simulink model "Step_1_Observer_Calibration_Experiment"  (R2020a)
settings: Solver=ode4  StartTime=0.0  StopTime=3  FixedStep=1e-6  MaxStep=1e-4  RelTol=1e-3
libraries: fl_lib x5, nesl_utility x5, ee_lib x2, simulink x1, eePwmGenerator x1
settings Model: Creator=nnnmmm  LastModifiedBy=nnnmmm
settings DataIOCC: ExternalInput=sim_input_T

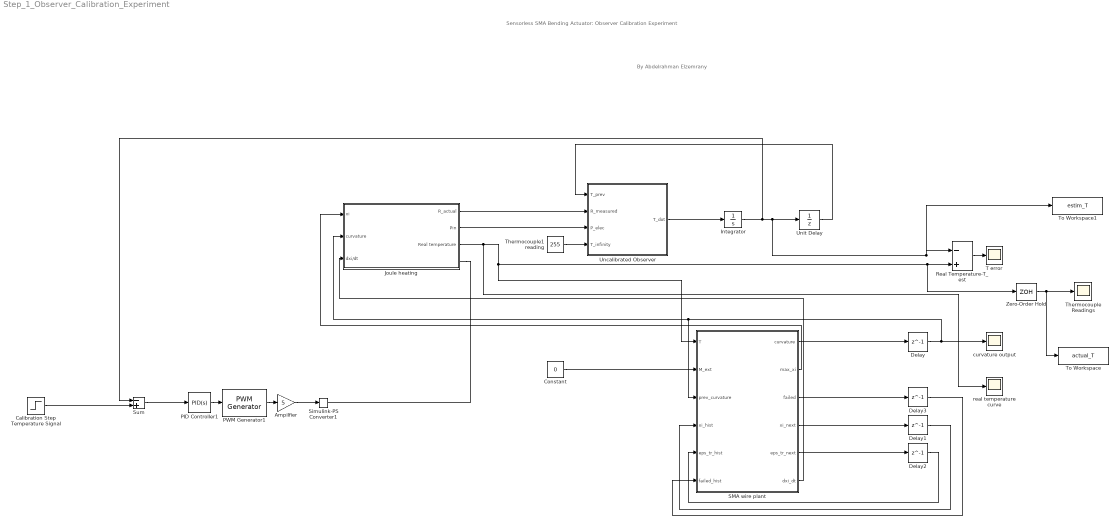
== system Step_1_Observer_Calibration_Experiment ==
  note: By Abdelrahman Elzemrany
  note: Sensorless SMA Bending Actuator: Observer Calibration Experiment
  Ampilfier : Gain  Gain=5
  Calibration Step Temperature Signal : Step  Before=255  After=300  SampleTime=0
  Constant : Constant  Value=0
  Delay : Delay  DelayLength=1
  Delay1 : Delay  DelayLength=1  InitialCondition=ones(1,11)
  Delay2 : Delay  DelayLength=1  InitialCondition=zeros(1,11)
  Delay3 : Delay  DelayLength=1
  Integrator : Integrator  InitialCondition=255
  Joule heating : Subsystem
  PID Controller1 : simulink/Continuous/PID Controller  Controller=PID  Form=Parallel  TimeDomain=Continuous-time  UseExternalTs=off  SampleTime=-1  IntegratorMethod=Forward Euler  FilterMethod=Forward Euler  ControllerParametersSource=internal  P=10  I=5  D=0  UseFilter=on  N=100  TunerSelectOption=Transfer Function Based (PID Tuner App)  InitialConditionSource=internal  InitialConditionForIntegrator=0  InitialConditionForFilter=0  DifferentiatorICPrevScaledInput=0  ExternalReset=none  TrackingMode=off  Kt=1  LimitOutput=on  UpperSaturationLimit=1  LowerSaturationLimit=0  LinearizeAsGain=on  AntiWindupMode=clamping  Kb=1  POutMin=[]  POutMax=[]  IOutMin=[]  IOutMax=[]  DOutMin=[]  DOutMax=[]  NOutMin=[]  NOutMax=[]  SumOutMin=[]  SumOutMax=[]  SaturationOutMin=[]  SaturationOutMax=[]  PParamMin=[]  PParamMax=[]  IParamMin=[]  IParamMax=[]  DParamMin=[]  DParamMax=[]  NParamMin=[]  NParamMax=[]  KbParamMin=[]  KbParamMax=[]  KtParamMin=[]  KtParamMax=[]  KbOutMin=[]  KbOutMax=[]  KtOutMin=[]  KtOutMax=[]  IntegratorOutMin=[]  IntegratorOutMax=[]  FilterOutMin=[]  FilterOutMax=[]  SumI1OutMin=[]  SumI1OutMax=[]  SumI2OutMin=[]  SumI2OutMax=[]  SumI3OutMin=[]  SumI3OutMax=[]  SumI4OutMin=[]  SumI4OutMax=[]  SumDOutMin=[]  SumDOutMax=[]  DifferentiatorOutMin=[]  DifferentiatorOutMax=[]  FilterDiffOutCoefMin=[]  FilterDiffOutCoefMax=[]  ReciprocalOutMin=[]  ReciprocalOutMax=[]  SumDenOutMin=[]  SumDenOutMax=[]  SumNumOutMin=[]  SumNumOutMax=[]  DivideOutMin=[]  DivideOutMax=[]  UdiffTsProdOutMin=[]  UdiffTsProdOutMax=[]  NTsProdOutMin=[]  NTsProdOutMax=[]  UintegralTsProdOutMin=[]  UintegralTsProdOutMax=[]  UngainTsProdOutMin=[]  UngainTsProdOutMax=[]  IntegratorContinuousStateAttributes=''  IntegratorStateMustResolveToSignalObject=off  IntegratorRTWStateStorageClass=Auto  FilterContinuousStateAttributes=''  FilterStateMustResolveToSignalObject=off  FilterRTWStateStorageClass=Auto  ParallelPVariant=InternalParameters  IdealPVariant=Disabled  IVariant=InternalParameters  DVariant=InternalParameters  IntegratorVariant=Continuous  SatVariant=Enabled  AWVariant=ContClampingParallel  PCopyVariant=Disabled  TRVariant=Disabled  FdbkBlocksVariant=Forward  IdealPFdbkVariant=Disabled  SatFdbkVariant=Disabled  DerivativeFilterVariant=ContFilter  NVariant=InternalParameters  NCopyVariant=Disabled  FilterICVariant=InternalICsFilter  IntegratorICVariant=InternalICs  ExternalResetVariant=Disabled  TRSumVariant=Passthrough  SumFdbkVariant=Disabled  SumVariant=Sum_PID  TsampFilterVariant=InternalTs  TsampNgainVariant=Passthrough  TsampIntegralVariant=Passthrough
  PWM Generator1 : eePwmGenerator/PWM Generator  CarrCount=Up  Tper=.00001  Ts=1e-6
  Real Temperature-T_est : Sum  Inputs=|-+
  SMA wire plant : MATLAB Function  TreatAsAtomicUnit=on
  Simulink-PS Converter1 : nesl_utility/Simulink-PS Converter  PhysicalDomain=network_engine_domain  SubClassName=ps_input  LeftPortType=input  RightPortType=output  PseudoPeriodic=off  Frequencies=[]  NoiseDistribution=none  NoiseParameters=[]  Unit=1  AffineConversion=off  FilteringAndDerivatives=filter  SimscapeFilterOrder=1  InputFilterTimeConstant=1e-6  UdotUserProvided=0
  Sum : Sum  Inputs=-+
  T error : Scope
  Thermocouple Readings : Scope
  Thermocouple1 reading : Constant  Value=255
  To Workspace : ToWorkspace  VariableName=actual_T  SaveFormat=Timeseries  SampleTime=.230
  To Workspace1 : ToWorkspace  VariableName=estim_T  SaveFormat=Timeseries  SampleTime=.001
  Uncalibrated Observer : MATLAB Function  TreatAsAtomicUnit=on
  Unit Delay : UnitDelay  SampleTime=-1  HasFrameUpgradeWarning=on
  Zero-Order Hold : ZeroOrderHold  SampleTime=.230
  curvature output : Scope
  real temperature curve : Scope
  wires:
  Delay2/1 -> SMA wire plant/5(eps_tr_hist)
  SMA wire plant/5(eps_tr_next) -> Delay2/1
  SMA wire plant/1(curvature) -> Delay/1
  SMA wire plant/3(failed) -> Delay3/1
  SMA wire plant/4(xi_next) -> Delay1/1
  Delay/1 -> curvature output/1, Joule heating/2(curvature), SMA wire plant/3(prev_curvature)
  Delay3/1 -> SMA wire plant/6(failed_hist)
  Delay1/1 -> SMA wire plant/4(xi_hist)
  Constant/1 -> SMA wire plant/2(M_ext)
  SMA wire plant/2(max_xi) -> Joule heating/1(xi)
  SMA wire plant/6(dxi_dt) -> Joule heating/3(dxi/dt)
  PWM Generator1/1 -> Ampilfier/1
  PID Controller1/1 -> PWM Generator1/1
  Ampilfier/1 -> Simulink-PS Converter1/1
  Joule heating/2(Pin) -> Uncalibrated Observer/3(P_elec)
  Joule heating/1(R_actual) -> Uncalibrated Observer/2(R_measured)
  Uncalibrated Observer/1(T_dot) -> Integrator/1
  Integrator/1 -> Sum/1, Unit Delay/1, To Workspace1/1, Real Temperature-T_est/1
  Thermocouple1 reading/1 -> Uncalibrated Observer/4(T_infinity)
  Joule heating/3(Real temperature) -> real temperature curve/1, SMA wire plant/1(T), Zero-Order Hold/1, Real Temperature-T_est/2
  Real Temperature-T_est/1 -> T error/1
  Unit Delay/1 -> Uncalibrated Observer/1(T_prev)
  Sum/1 -> PID Controller1/1
  Calibration Step Temperature Signal/1 -> Sum/2
  Zero-Order Hold/1 -> To Workspace/1, Thermocouple Readings/1
  connections:
  Joule heating/RConn1 -- Simulink-PS Converter1/RConn1

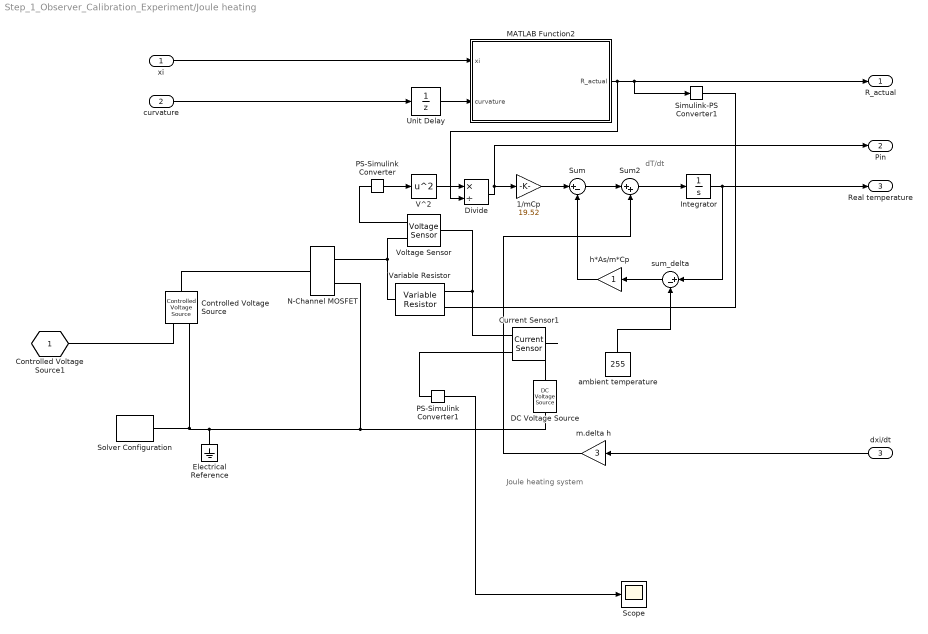
== system Step_1_Observer_Calibration_Experiment/Joule heating ==
  note: Joule heating system
  note: dT/dt
  xi : Inport
  curvature : Inport  Port=2
  dxi/dt : Inport  Port=3
  1/mCp : Gain  Gain=19.52
  Controlled Voltage Source : fl_lib/Electrical/Electrical Sources/Controlled Voltage Source
  Current Sensor1 : fl_lib/Electrical/Electrical Sensors/Current Sensor
  DC Voltage Source : ee_lib/Additional Components/SPICE Sources/DC Voltage Source  DC=2 V
  Divide : Product  Inputs=*/
  Electrical Reference : fl_lib/Electrical/Electrical Elements/Electrical Reference
      settings: SourceProductBaseCode=MT,SS
  Integrator : Integrator  InitialCondition=255
  MATLAB Function2 : MATLAB Function  TreatAsAtomicUnit=on
  N-Channel MOSFET : ee_lib/Semiconductors & Converters/N-Channel MOSFET  paramTerminal=ee.enum.mosfet.numberOfTerminals.three  parameterization=ee.enum.parameterization.datasheet  prmDatasheet=ee.enum.temperatureParameterization.none  prmEquCoeff=ee.enum.temperatureParameterization.none  Beta=5.0 A/V^2  Rds=0.010 Ohm  Id=6.0 A  Vgs=10 V  Vth=1.7 V  Vth0=1.7 V  lam=0 1/V  gamma_vth=0.5 V^0.50000  phib=0.5 V  Vth1=1.9071 V  Vbs1=-1 V  Vth2=2.066 V  Vbs2=-2 V  Tmeas=25 degC  RS=0.0001 Ohm  RD=1e-4 Ohm  RB=0.001 Ohm  C_param=ee.enum.mosfet.capacitanceParam.fixedciss  C_GS=270 pF  C_GD=80 pF  C_DS=0 pF  C_iss=350 pF  C_rss=80 pF  C_oss=0 pF  charge_linearity_param=ee.enum.mosfet.cgdLinearity.constant  C_OX=200 pF  V_C_OX=-0.5 V  C_iss_vec=[720, 700, 590, 470, 390, 310] pF  C_rss_vec=[450, 400, 300, 190, 95, 55] pF  C_oss_vec=[900, 810, 690, 420, 270, 170] pF  C_GS_vec=[270, 300, 290, 280, 295, 255] pF  C_GD_vec=[450, 400, 300, 190, 95, 55] pF  C_DS_vec=[450, 410, 390, 230, 175, 115] pF  C_Vds_vec=[.1, .3, 1, 3, 10, 30] V  V_GS_for_cap_data=0 V  charge_linearity_param_vgb=ee.enum.mosfet.cgbLinearity.instantly  IsDiode=0 A  Vbi=0.6 V  n=1  Cj0Diode=0 pF  TT=50e-9 s  dVth_dT=-6 mV/K  dVth0_dT=-6 mV/K  Rds_T2=0.037 Ohm  Tmeas2=125 degC  BEXDatasheet=-1.5  BEXEquCoeff=-1.5  etaisDatasheet=3  etaisEquCoeff=3  TdeviceDatasheet=25 degC  TdeviceEquCoeff=25 degC  thermal_network_parameterization=ee.enum.thermalNetworkTopology.cauer  Rth=[0, 10] K/W  Rth_Foster=[4, 6] K/W  thermal_mass_parameterization=ee.enum.thermalNetwork.timeconstant  thermal_mass=[0, 1] J/K  thermal_mass_Foster=[1.5, 3] J/K  thermal_time_constant=[0, 10] s  thermal_time_constant_Foster=[6, 18] s  thermal_mass_initial_temperatures=[25, 25] degC  betaref=18 A/V^2  Vfbref=-1.1 V  gamma=3.5 V^0.50000  phib2ref=1 V  thesatref=0.4 1/V  alpha=0  Vp=5e-2 V  thesrref=0 1/V  m=8  Tref=25 degC  Cox=1500 pF  Cgso=100 pF  Cgdo=14 pF  Rsref=2e-3 Ohm  Rdref=0.17 Ohm  Rgref=8.4 Ohm  Rbref=2e-3 Ohm  Isref=5.2e-13 A  Cj0=480 pF  Tprm=1  etabet=1.3  Stvfb=5e-4 V/K  Stphib=-8.5e-4 V/K  etasat=1.04  etasr=0.65  etar=0.95  etais=3  Tsim=25 degC  T0=[25, 25] degC
  PS-Simulink Converter : nesl_utility/PS-Simulink Converter  PhysicalDomain=network_engine_domain  SubClassName=ps_output  LeftPortType=input  RightPortType=output  PseudoPeriodic=off  Frequencies=[]  Unit=inherit  AffineConversion=off
  PS-Simulink Converter1 : nesl_utility/PS-Simulink Converter  PhysicalDomain=network_engine_domain  SubClassName=ps_output  LeftPortType=input  RightPortType=output  PseudoPeriodic=off  Frequencies=[]  Unit=inherit  AffineConversion=off
  Scope : Scope
  Simulink-PS Converter1 : nesl_utility/Simulink-PS Converter  PhysicalDomain=network_engine_domain  SubClassName=ps_input  LeftPortType=input  RightPortType=output  PseudoPeriodic=off  Frequencies=[]  NoiseDistribution=none  NoiseParameters=[]  Unit=1  AffineConversion=off  FilteringAndDerivatives=provide  SimscapeFilterOrder=1  InputFilterTimeConstant=0.001  UdotUserProvided=0
  Solver Configuration : nesl_utility/Solver Configuration  PhysicalDomain=network_engine_domain  SubClassName=solver  LeftPortType=input  RightPortType=generic  Tones=[]  Harmonics=[]  SimulateNoise=off  Profile=off  UseLocalSampling=off  EnableSwitchedLinearOptims=on  FrequencyDomain=off  UseCCode=off  RelTol=0.001  AbsTol=1e-06  MinStep=1e-09  ToWorkspace=off  RevertToSquareIcSolve=off  NumHomotopyIterations=100  PhasorMode=off  PhasorModeNumHarmonics=1  DoDC=off  ResidualTolerance=1e-09  UseLocalSolver=on  LocalSolverChoice=NE_BACKWARD_EULER_ADVANCER  LocalSolverSampleTime=1e-3  DoFixedCost=on  MaxNonlinIter=20  MaxModeIter=2  LinearAlgebra=auto  EquationFormulation=NE_TIME_EF  DelaysMemoryBudget=1024  AutomaticFiltering=on  FilteringTimeConstant=0.001  PartitionStorageMethod=AS_NEEDED  PartitionMemoryBudget=1024  PartitionMethod=ROBUST
  Sum : Sum  Inputs=|+-
  Sum2 : Sum  Inputs=|++
  Unit Delay : UnitDelay  SampleTime=-1  HasFrameUpgradeWarning=on
  V^2 : Math  Operator=square  SaturateOnIntegerOverflow=on
  Variable Resistor : fl_lib/Electrical/Electrical Elements/Variable Resistor  Rmin=0 Ohm  i_specify=off  i_priority=None  i=0 A  i_nominal_specify=off  i_nominal_unit=A  i_nominal_value=1  v_specify=off  v_priority=None  v=0 V  v_nominal_specify=off  v_nominal_unit=V  v_nominal_value=1
  Voltage Sensor : fl_lib/Electrical/Electrical Sensors/Voltage Sensor
  ambient temperature : Constant  Value=255
  h*As/m*Cp : Gain
  m.delta h : Gain  Gain=3
  sum_delta : Sum  Inputs=|+-
  Controlled Voltage Source1 : PMIOPort  Side=Right
  R_actual : Outport
  Pin : Outport  Port=2
  Real temperature : Outport  Port=3
  wires:
  Integrator/1 -> Real temperature/1, sum_delta/1
  1/mCp/1 -> Sum/1
  Sum/1 -> Sum2/1
  Sum2/1 -> Integrator/1
  PS-Simulink Converter/1 -> V^2/1
  ambient temperature/1 -> sum_delta/2
  V^2/1 -> Divide/1
  h*As/m*Cp/1 -> Sum/2
  sum_delta/1 -> h*As/m*Cp/1
  m.delta h/1 -> Sum2/2
  Divide/1 -> Pin/1, 1/mCp/1
  MATLAB Function2/1(R_actual) -> Divide/2, R_actual/1, Simulink-PS Converter1/1
  dxi/dt/1 -> m.delta h/1
  curvature/1 -> Unit Delay/1
  Unit Delay/1 -> MATLAB Function2/2(curvature)
  xi/1 -> MATLAB Function2/1(xi)
  PS-Simulink Converter1/1 -> Scope/1
  connections:
  Solver Configuration/RConn1 -- Electrical Reference/LConn1 -- DC Voltage Source/RConn1 -- N-Channel MOSFET/RConn2 -- Controlled Voltage Source/RConn2
  N-Channel MOSFET/RConn1 -- Variable Resistor/RConn1 -- Voltage Sensor/RConn2
  Simulink-PS Converter1/RConn1 -- Variable Resistor/LConn1
  Voltage Sensor/LConn1 -- Current Sensor1/RConn2 -- Variable Resistor/LConn2
  Controlled Voltage Source/LConn1 -- N-Channel MOSFET/LConn1
  Voltage Sensor/RConn1 -- PS-Simulink Converter/LConn1
  Current Sensor1/RConn1 -- PS-Simulink Converter1/LConn1
  Current Sensor1/LConn1 -- DC Voltage Source/LConn1
  Controlled Voltage Source/RConn1 -- Controlled Voltage Source1/RConn1

== matlab function Step_1_Observer_Calibration_Experiment/SMA wire plant ==
  data: T input; M_ext input; prev_curvature input; xi_hist input; eps_tr_hist input; curvature output; max_xi output; failed_hist input; failed output; xi_next output; eps_tr_next output; dxi_dt output
function [curvature, max_xi,  failed, xi_next, eps_tr_next, dxi_dt] = lagoudas_wire_pure_bending(T , M_ext, prev_curvature, xi_hist, eps_tr_hist, failed_hist)
%#codegen

% =========================================================================
% ─── SIMULINK CODER INCLUSIONS: IMMEDIATE VARIABLE INITIALIZATION ───
% =========================================================================
failed = failed_hist; % FIX: Inherit historical failure state immediately
curvature = prev_curvature;
max_xi = 0.0;
surface_sigma = 0.0;
dxi_dt = 0.0; 

% Strict [11 x 1] column vector properties for code generation alignment
xi_next = zeros(11, 1);
eps_tr_next = zeros(11, 1);

% Early exit if the wire has already failed historically
if failed_hist > 0.5
    failed = 1.0;
    return;
end

% =========================================================================
% 1. WIRE CROSS-SECTIONAL SLICE DISCRETIZATION (11 Symmetrical Layers)
% =========================================================================
R_wire = 0.25e-3;   
N_layers = 11;      
y_coords = linspace(-R_wire, R_wire, N_layers); 
y_coords = y_coords(:); 
dy = y_coords(2) - y_coords(1);
dt = 0.0001;        

xi_current = xi_hist(:);
eps_tr_current = eps_tr_hist(:);

% =========================================================================
% 2. EXPLICIT MATERIAL LITERAL CONSTANTS
% =========================================================================
E_A = 70e9;             
E_M = 30e9;             
H_max = 0.045;          
sigma_failure = 1000e6; 

Ms = 275; Mf = 263; As = 280; Af = 300; % Ms updated to 280 K
C_A = 8e6; C_M = 8e6;   
n1 = 2.0; n2 = 2.0; n3 = 2.0; n4 = 2.0; 

S_A = 1 / E_A; S_M = 1 / E_M; Delta_S = S_M - S_A; 

w_layer = 2 * sqrt(max(0, R_wire^2 - y_coords.^2));
dA = w_layer * dy;
S_curr_static = S_A + xi_current * Delta_S;

% =========================================================================
% 3. VECTORIZED EXPLICIT STATIC SOLVER LOOP FOR MECHANICAL EQUILIBRIUM
% =========================================================================
low_k = -150.0; 
high_k = 150.0; 
tol = 1e-6;
curvature = prev_curvature;
residual_mid = 0.0;

for iter = 1:60
    mid_k = (low_k + high_k) / 2;
    
    % Evaluate midpoint state residual
    eps_mid = -y_coords * mid_k;
    sigma_mid = (eps_mid - eps_tr_current) ./ S_curr_static;
    M_calc_mid = sum(-sigma_mid .* y_coords .* dA);
    residual_mid = M_calc_mid - M_ext;
    
    % Evaluate low-point state residual dynamically inside the loop
    % FIX: This forces the boundary checks to update with each step
    eps_low = -y_coords * low_k;
    sigma_low = (eps_low - eps_tr_current) ./ S_curr_static;
    M_calc_low = sum(-sigma_low .* y_coords .* dA);
    residual_low = M_calc_low - M_ext;
    
    if abs(residual_mid) < tol
        curvature = mid_k;
        break;
    end
    
    if (residual_low * residual_mid) < 0
        high_k = mid_k;
    else
        low_k = mid_k;
    end
end

if abs(residual_mid) >= tol
    curvature = (low_k + high_k) / 2;
end

% =========================================================================
% 4. LAYER PROGRESSION UPDATE WITH EXPLICIT RELAXATION FILTERING
% =========================================================================
sigma_max_track = 0.0;
xi_unfiltered = zeros(N_layers, 1);

for j = 1:N_layers
    epsilon = -y_coords(j) * curvature;
    S_curr = S_A + xi_current(j) * Delta_S;
    sigma_layer = (epsilon - eps_tr_current(j)) / S_curr;
    
    if abs(sigma_layer) > sigma_max_track
        sigma_max_track = abs(sigma_layer);
    end
    
    sgn_sig = sign(sigma_layer);
    if sgn_sig == 0; sgn_sig = 1; end
    
    Ms_s = Ms + abs(sigma_layer) / C_M;
    Mf_s = Mf + abs(sigma_layer) / C_M;
    As_s = As + abs(sigma_layer) / C_A;
    Af_s = Af + abs(sigma_layer) / C_A;
    
    xi_target = xi_current(j); 
    
    if abs(curvature) > 0.000
        if (T < Ms_s) && (T > Mf_s)
            linear_ratio = (T - Mf_s) / (Ms_s - Mf_s);
            trial_target = 1.0 - (linear_ratio^n1 / (linear_ratio^n1 + (1.0 - linear_ratio)^n2));
            if trial_target > xi_current(j); xi_target = trial_target; end
        elseif T <= Mf_s
            xi_target = 1.0;
        end
        
        if (T > As_s) && (T < Af_s)
            linear_ratio = (T - As_s) / (Af_s - As_s);
            trial_target = 1.0 - (linear_ratio^n3 / (linear_ratio^n3 + (1.0 - linear_ratio)^n4));
            if trial_target < xi_current(j); xi_target = trial_target; end
        elseif T >= Af_s
            xi_target = 0.0;
        end
    else
        if T > Af; xi_target = 0.0; elseif T < Mf; xi_target = 1.0; end
    end
    
    xi_unfiltered(j) = xi_target;
    
    % Balanced 5% relaxation factor
    xi_current(j) = xi_hist(j) + 0.05 * (xi_target - xi_hist(j));
    
    sigma_detwin = 70e6;
    if abs(sigma_layer) > 1e-3
        detwin_factor = min(1.0, abs(sigma_layer) / sigma_detwin);
        eps_tr_target = sgn_sig * H_max * xi_current(j) * detwin_factor;
    else
        eps_tr_target = 0.0;
    end
    
    eps_tr_current(j) = eps_tr_hist(j) + 0.05 * (eps_tr_target - eps_tr_hist(j));
end

if sigma_max_track > sigma_failure
    failed = 1.0;
end

% =========================================================================
% 5. ASSIGN FINAL OUTPUT PARAMETERS
% =========================================================================
max_xi = max(xi_current);
surface_sigma = sigma_max_track;

mean_xi_target = mean(xi_unfiltered);
mean_xi_hist = mean(xi_hist);
dxi_dt = (mean_xi_target - mean_xi_hist) / dt;

xi_next = xi_current(:);
eps_tr_next = eps_tr_current(:);

end

== matlab function Step_1_Observer_Calibration_Experiment/Joule heating/MATLAB Function2 ==
  data: xi input; R_actual output; curvature input
function R_actual = dynamic_resistance_block_final(xi, curvature)
%#codegen
% Final 0.5mm Wire Variant - Replaces the static .16 and .92 blocks.
% Driven directly by the model's curvature output.

%% 1. Fixed Mechanical & Nominal Parameters
r_wire  = 0.00025;    % Wire radius (0.5mm diameter = 0.25mm radius)

% 0.5mm Nominal Baseline Boundaries (Adjust based on your wire length)
Rm_base = 1.08;      % Cold Martensite baseline resistance boundary
Ra_base = 0.92;      % Hot Austenite baseline resistance boundary

% Material Piezoresistive Gauge Coefficients
K_a = 2.15;           % Hot phase gauge factor
K_m = 1.90;           % Cold phase gauge factor

%% 2. Direct Strain Conversion from Curvature
epsilon = curvature * r_wire;

% Bounds check to prevent numerical instability outside valid physical strain limits
if epsilon < 0.0, epsilon = 0.0; end
if epsilon > 0.06, epsilon = 0.06; end % Cap at 6% maximum strain 

%% 3. Dynamic Boundary Scaling Matrix
Ra_dynamic = Ra_base * (1 + K_a * epsilon);
Rm_dynamic = Rm_base * (1 + K_m * epsilon);

delta_R_dynamic = Rm_dynamic - Ra_dynamic;

% --- REPRODUCING YOUR BLOCKS ---
% Replicates: (xi * Delta_R) + Ra_base
R_actual = (xi * delta_R_dynamic) + Ra_dynamic;

end

== matlab function Step_1_Observer_Calibration_Experiment/Uncalibrated Observer ==
  settings: updateMethod=DISCRETE
  data: T_prev input; R_measured input; P_elec input; T_dot output; T_infinity input
function T_dot  = sma_thermal_observer(T_prev,R_measured,P_elec ,  T_infinity)
%#codegen
% Corrected Continuous Sensorless Thermal Observer for SMA Wire
% Inputs: 
%   P_elec      = Real-time electrical power from measurement block (Watts)
%   R_measured  = Real-time resistance from measurement block (Ohms)
%   T_prev      = Fed-back estimated temperature from the last step (Kelvin)
%   T_infinity  = Ambient baseline temperature (255 Kelvin)
% Outputs:
%   T_dot       = Rate of temperature change (dT/dt) to feed your Integrator
%   xi          = Calculated Martensite Volume Fraction state

%% 1. Physical Parameter Constants (0.25g Mass Alignment)
m_wire   = 0.0001276;         % Wire Mass: Exact 0.25 grams -> 0.00025 kg
Cp       =  410    ;           % Specific Heat Capacity: 400 J/kg.K
h        =  326.8  ;           % Convective Heat Transfer Coeff: 515 W/m^2.K
As       = 1.5708e-4;       % Wire Surface Area: 1.5708 * 10^-4 m^2
latent_H = 22000.0;         % Latent heat of transformation enthalpy (J/kg)

% Pre-calculate denominators to optimize execution speed
m_Cp = m_wire * Cp;         % Thermal Inertia denominator (0.1)
h_As = h * As;              % Environmental cooling gain constant

%% 2. Process Environmental Thermal Loss
P_loss = h_As * (T_prev - T_infinity);

%% 3. Continuous Observer Decision Logic
persistent xi_prev;
if isempty(xi_prev)
    xi_prev = 1.0;          % Initialize at 100% Martensite
end

% Linearly map the Martensite Volume Fraction (xi) directly across your entire resistance profile
% 1.08 Ohms = 100% Martensite (xi = 1.0) | 0.92 Ohms = 0% Martensite (xi = 0.0)
xi = (R_measured - 0.92) / (1.08 - 0.92);

% Strictly bound xi between 0 (fully Austenite) and 1 (fully Martensite)
if xi > 1.0, xi = 1.0; end
if xi < 0.0, xi = 0.0; end

% Approximate the discrete rate of transformation change (dXi/dt)
dt_step = 0.001;        % Fixed sample interval matching your 1ms controller rate
dXi_dt = (xi - xi_prev) / dt_step;

% Calculate latent heat transformation load
P_latent = m_wire * latent_H * dXi_dt;

% --- SINGLE UNIFIED PHYSICS EQUATION ---
% No hard stalls at 280K. If the wire is pre-switch, xi will naturally be 1.0,
% meaning dXi_dt will be 0, and P_latent turns off automatically!
T_dot = (P_elec - P_loss - P_latent) / m_Cp;

% Update memory buffer for next time frame step
xi_prev = xi;
